simulink model "Model_Simulation"  (R2016a)
settings: Solver=FixedStepAuto  StartTime=0.0  StopTime=5  FixedStep=2e-6  RelTol=1e-3
values from neighbouring files (symbols this model uses):
  C = 3060e-6    (= 0.00306)    [Controle_Inversor_UR_D.m]
  Ki_i_disc = wc*Rf    (= 44.2477838534)    [Controle_Inversor_UR_D.m]
  Ki_i_disc_b = wc_b*Rb/Vdc    (= 0.0983284085631)    [Controle_Inversor_UR_D.m]
  Ki_q_disc = wq/H    [Controle_Inversor_UR_D.m]
  Ki_v_disc_b = wc_bv/Req    (= 14.5799013102)    [Controle_Inversor_UR_D.m]
  Ki_vdc_disc = ((wvdc)^2*C)/Gt    [Controle_Inversor_UR_D.m]
  Kp_i_disc = wc*Lf    (= 2.19688771906)    [Controle_Inversor_UR_D.m]
  Kp_i_disc_b = wc_b*Lb/Vdc    (= 0.00545604673435)    [Controle_Inversor_UR_D.m]
  Kp_q_disc = Ki_q_disc*(Lf/Kp_i_disc)    [Controle_Inversor_UR_D.m]
  Kp_v_disc_b = wc_bv*Cin    (= 0.0356301510224)    [Controle_Inversor_UR_D.m]
  Kp_vdc_disc = (2*ksi_vdc*wvdc*C)/Gt    [Controle_Inversor_UR_D.m]
  Lf = (0.0012+2.8949e-04)    (= 0.00148949)    [Controle_Inversor_UR_D.m]
  Tsw = 1/fsw    (= 0.0002)    [Controle_Inversor_UR_D.m]
  w = 2*pi*60    (= 376.991118431)    [Controle_Inversor_UR_D.m]
undefined symbols (not defined in the file or in its folder): D1, dEgdT, Delta, EgRef, gcbh, k1, Rsh_array5pc, sigbuilder_block, sps_rtmsupport, Tref_K, VT_ref
libraries: powerlib x179, simulink x14, powerlib_meascontrol x13, spsPVarrayModel x12
(part 20 of 20)

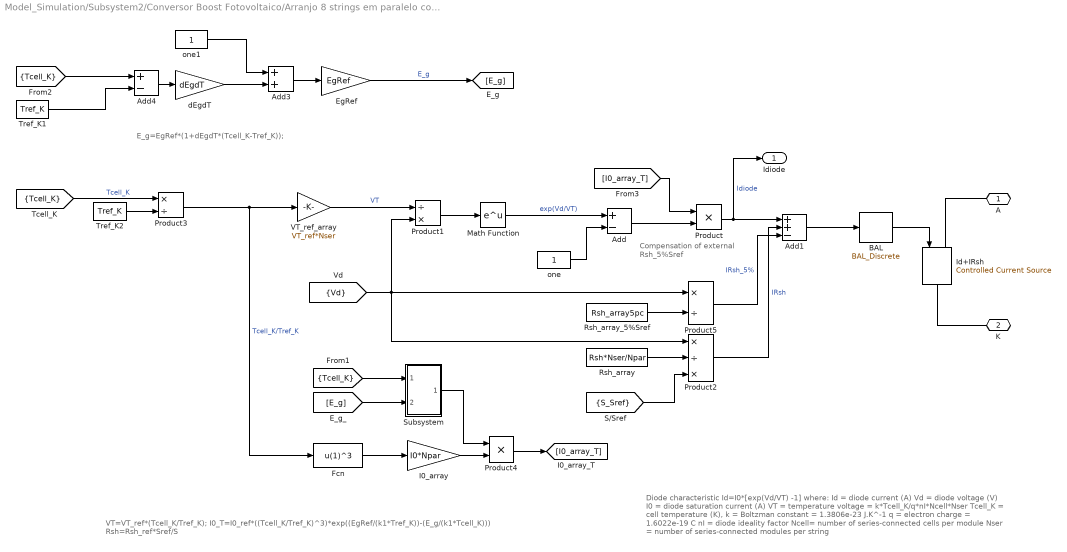
== system Model_Simulation/Subsystem2/Conversor Boost Fotovoltaico/Arranjo 8 strings em paralelo com 43 módulos em série Vmp = 43 x 30,6 = 1315,8 V Imp = 8,32 x 7 = 58,24 A 76.632,192 W/Diode Rsh ==
  note: E_g=EgRef*(1+dEgdT*(Tcell_K-Tref_K));
  note: VT=VT_ref*(Tcell_K/Tref_K);
      | I0_T=I0_ref*((Tcell_K/Tref_K)^3)*exp((EgRef/(k1*Tref_K))-(E_g/(k1*Tcell_K)))
      | Rsh=Rsh_ref*Sref/S
  note: Diode characteristic
      |    Id=I0*[exp(Vd/VT) -1]
      |
      | where:
      |      Id = diode current (A)
      |      Vd = diode voltage (V)
      |      I0 = diode saturation current (A)
      |      VT = temperature voltage = k*Tcell_K/q*nI*Ncell*Nser
      | Tcell_K = cell temperature (K),
      |       k = Boltzman constant = 1.3806e-23 J.K^-1
      |       q = electron charge = 1.6022e-19 C
      |      nI = diode ideality factor
      |    Ncell= number of series-connected cells per module
      |    Nser = number of series-connected modules per string
  note: Compensation of
      | external Rsh_5%Sref
  Add : Sum  Inputs=+-
  Add1 : Sum  Inputs=++-
  Add3 : Sum
  Add4 : Sum  Inputs=+-
  BAL : spsPVarrayModel/BAL_Discrete  VariantControl=NoBAL
  EgRef : Gain  Gain=EgRef
  Fcn : Fcn  Expr=u(1)^3
  I0_array : Gain  Gain=I0*Npar
  Id+IRsh : powerlib/Electrical Sources/Controlled Current Source  Initialize=on  Source_Type=AC  Amplitude=0  Phase=0  Frequency=0  Measurements=None
  Math Function : Math  SaturateOnIntegerOverflow=on
  Product : Product  RndMeth=Zero
  Product1 : Product  Inputs=/*  RndMeth=Zero
  Product2 : Product  Inputs=*/*  RndMeth=Zero
  Product3 : Product  Inputs=*/  RndMeth=Zero
  Product4 : Product  Inputs=**  RndMeth=Zero
  Product5 : Product  Inputs=*/  RndMeth=Zero
  Rsh_array : Constant  Value=Rsh*Nser/Npar
  Rsh_array_5%Sref : Constant  Value=Rsh_array5pc
  Subsystem : Subsystem
  Tref_K1 : Constant  Value=Tref_K
  Tref_K2 : Constant  Value=Tref_K
  VT_ref_array : Gain  Gain=VT_ref*Nser
  dEgdT : Gain  Gain=dEgdT
  one : Constant
  one1 : Constant
  A : PMIOPort  Port=1  Side=Left
  K : PMIOPort  Port=2  Side=Right
  Idiode : Outport
  wires:
  [Vd] -> Product1/2, Product2/1, Product5/1
  [S_Sref] -> Product2/3
  [I0_array_T] -> Product/1
  VT_ref_array/1 -> Product1/1  "VT"
  Add/1 -> Product/2
  Product4/1 -> [I0_array_T]
  Tref_K2/1 -> Product3/2
  [E_g] -> Subsystem/2(E_g)
  [Tcell_K] -> Subsystem/1(Tcell_K)
  Subsystem/1(exp) -> Product4/1
  Tref_K1/1 -> Add4/2
  [Tcell_K] -> Add4/1
  Fcn/1 -> I0_array/1
  I0_array/1 -> Product4/2
  EgRef/1 -> [E_g]  "E_g"
  Add3/1 -> EgRef/1
  dEgdT/1 -> Add3/2
  Add4/1 -> dEgdT/1
  one1/1 -> Add3/1
  Product3/1 -> Fcn/1, VT_ref_array/1  "Tcell_K/Tref_K"
  [Tcell_K] -> Product3/1  "Tcell_K"
  Rsh_array/1 -> Product2/2
  one/1 -> Add/2
  Product1/1 -> Math Function/1
  Product/1 -> Idiode/1, Add1/1  "Idiode"
  Product2/1 -> Add1/2  "IRsh"
  Math Function/1 -> Add/1  "exp(Vd/VT)"
  Rsh_array_5%Sref/1 -> Product5/2
  Product5/1 -> Add1/3  "IRsh_5%"
  Add1/1 -> BAL/1
  BAL/1 -> Id+IRsh/1
  connections:
  A/RConn1 -- Id+IRsh/LConn1
  Id+IRsh/RConn1 -- K/RConn1

== system Model_Simulation/Subsystem2/Conversor Boost Fotovoltaico/Arranjo 8 strings em paralelo com 43 módulos em série Vmp = 43 x 30,6 = 1315,8 V Imp = 8,32 x 7 = 58,24 A 76.632,192 W/IL ctrl ==
  note: IL=S/Sref*(IL_ref+alpha_isc*(Tcell_K-Tref_K));
  Temperature : Inport
  Irradiance : Inport  Port=2
  0_K : Constant  Value=273.15
  1/Sref : Gain  Gain=1e-3
  Add : Sum
  Add2 : Sum
  Add3 : Sum  Inputs=+-
  IL_module : Constant  Value=IL
  Npar : Gain  Gain=Npar
  Product1 : Product  Inputs=**  RndMeth=Zero
  Tref_K : Constant  Value=Tref_K
  alpha_Isc : Gain  Gain=alpha_Isc
  IL : Outport
  tag scope: S_Sref=scoped, Tcell_K=scoped
  wires:
  1/Sref/1 -> [S_Sref], Product1/2  "S/Sref"
  Npar/1 -> Product1/1
  Add2/1 -> [Tcell_K], Add3/1  "Tcell_K"
  Add/1 -> Npar/1
  0_K/1 -> Add2/2
  IL_module/1 -> Add/2
  Product1/1 -> IL/1  "IL"
  Tref_K/1 -> Add3/2
  Add3/1 -> alpha_Isc/1
  alpha_Isc/1 -> Add/1
  Irradiance/1 -> 1/Sref/1
  Temperature/1 -> Add2/1

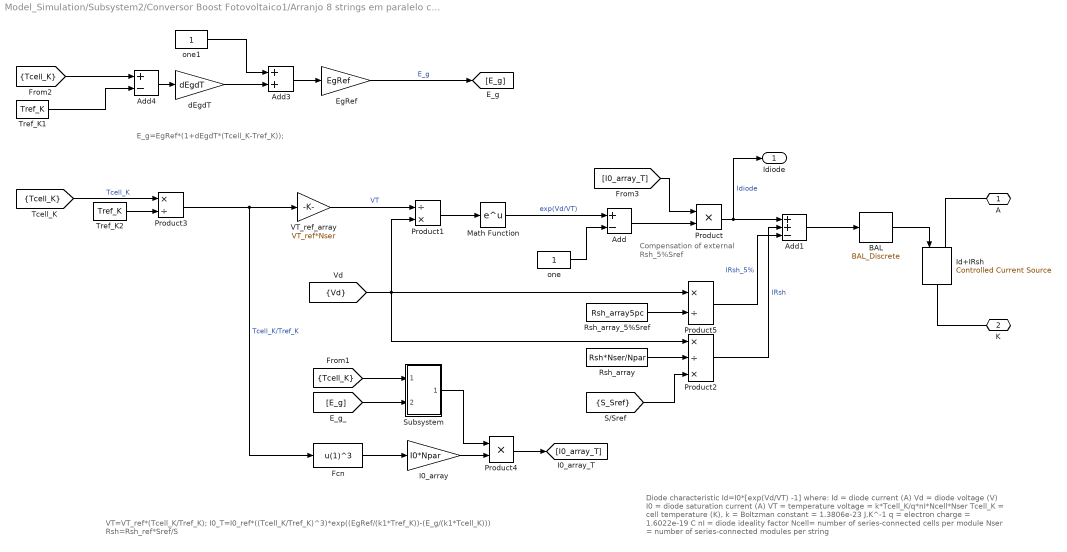
== system Model_Simulation/Subsystem2/Conversor Boost Fotovoltaico1/Arranjo 8 strings em paralelo com 43 módulos em série Vmp = 43 x 30,6 = 1315,8 V Imp = 8,32 x 7 = 58,24 A 76.632,192 W/Diode Rsh ==
  note: Compensation of
      | external Rsh_5%Sref
  note: Diode characteristic
      |    Id=I0*[exp(Vd/VT) -1]
      |
      | where:
      |      Id = diode current (A)
      |      Vd = diode voltage (V)
      |      I0 = diode saturation current (A)
      |      VT = temperature voltage = k*Tcell_K/q*nI*Ncell*Nser
      | Tcell_K = cell temperature (K),
      |       k = Boltzman constant = 1.3806e-23 J.K^-1
      |       q = electron charge = 1.6022e-19 C
      |      nI = diode ideality factor
      |    Ncell= number of series-connected cells per module
      |    Nser = number of series-connected modules per string
  note: VT=VT_ref*(Tcell_K/Tref_K);
      | I0_T=I0_ref*((Tcell_K/Tref_K)^3)*exp((EgRef/(k1*Tref_K))-(E_g/(k1*Tcell_K)))
      | Rsh=Rsh_ref*Sref/S
  note: E_g=EgRef*(1+dEgdT*(Tcell_K-Tref_K));
  Add : Sum  Inputs=+-
  Add1 : Sum  Inputs=++-
  Add3 : Sum
  Add4 : Sum  Inputs=+-
  BAL : spsPVarrayModel/BAL_Discrete  VariantControl=NoBAL
  EgRef : Gain  Gain=EgRef
  Fcn : Fcn  Expr=u(1)^3
  I0_array : Gain  Gain=I0*Npar
  Id+IRsh : powerlib/Electrical Sources/Controlled Current Source  Initialize=on  Source_Type=AC  Amplitude=0  Phase=0  Frequency=0  Measurements=None
  Math Function : Math  SaturateOnIntegerOverflow=on
  Product : Product  RndMeth=Zero
  Product1 : Product  Inputs=/*  RndMeth=Zero
  Product2 : Product  Inputs=*/*  RndMeth=Zero
  Product3 : Product  Inputs=*/  RndMeth=Zero
  Product4 : Product  Inputs=**  RndMeth=Zero
  Product5 : Product  Inputs=*/  RndMeth=Zero
  Rsh_array : Constant  Value=Rsh*Nser/Npar
  Rsh_array_5%Sref : Constant  Value=Rsh_array5pc
  Subsystem : Subsystem
  Tref_K1 : Constant  Value=Tref_K
  Tref_K2 : Constant  Value=Tref_K
  VT_ref_array : Gain  Gain=VT_ref*Nser
  dEgdT : Gain  Gain=dEgdT
  one : Constant
  one1 : Constant
  A : PMIOPort  Port=1  Side=Left
  K : PMIOPort  Port=2  Side=Right
  Idiode : Outport
  wires:
  BAL/1 -> Id+IRsh/1
  Add1/1 -> BAL/1
  Product5/1 -> Add1/3  "IRsh_5%"
  Rsh_array_5%Sref/1 -> Product5/2
  Math Function/1 -> Add/1  "exp(Vd/VT)"
  Product2/1 -> Add1/2  "IRsh"
  Product/1 -> Add1/1, Idiode/1  "Idiode"
  Product1/1 -> Math Function/1
  one/1 -> Add/2
  Rsh_array/1 -> Product2/2
  [Tcell_K] -> Product3/1  "Tcell_K"
  Product3/1 -> VT_ref_array/1, Fcn/1  "Tcell_K/Tref_K"
  one1/1 -> Add3/1
  Add4/1 -> dEgdT/1
  dEgdT/1 -> Add3/2
  Add3/1 -> EgRef/1
  EgRef/1 -> [E_g]  "E_g"
  I0_array/1 -> Product4/2
  Fcn/1 -> I0_array/1
  [Tcell_K] -> Add4/1
  Tref_K1/1 -> Add4/2
  Subsystem/1(exp) -> Product4/1
  [Tcell_K] -> Subsystem/1(Tcell_K)
  [E_g] -> Subsystem/2(E_g)
  Tref_K2/1 -> Product3/2
  Product4/1 -> [I0_array_T]
  Add/1 -> Product/2
  VT_ref_array/1 -> Product1/1  "VT"
  [I0_array_T] -> Product/1
  [S_Sref] -> Product2/3
  [Vd] -> Product5/1, Product2/1, Product1/2
  connections:
  Id+IRsh/RConn1 -- K/RConn1
  A/RConn1 -- Id+IRsh/LConn1

== system Model_Simulation/Subsystem2/Conversor Boost Fotovoltaico1/Arranjo 8 strings em paralelo com 43 módulos em série Vmp = 43 x 30,6 = 1315,8 V Imp = 8,32 x 7 = 58,24 A 76.632,192 W/IL ctrl ==
  note: IL=S/Sref*(IL_ref+alpha_isc*(Tcell_K-Tref_K));
  Temperature : Inport
  Irradiance : Inport  Port=2
  0_K : Constant  Value=273.15
  1/Sref : Gain  Gain=1e-3
  Add : Sum
  Add2 : Sum
  Add3 : Sum  Inputs=+-
  IL_module : Constant  Value=IL
  Npar : Gain  Gain=Npar
  Product1 : Product  Inputs=**  RndMeth=Zero
  Tref_K : Constant  Value=Tref_K
  alpha_Isc : Gain  Gain=alpha_Isc
  IL : Outport
  tag scope: S_Sref=scoped, Tcell_K=scoped
  wires:
  Temperature/1 -> Add2/1
  Irradiance/1 -> 1/Sref/1
  alpha_Isc/1 -> Add/1
  Add3/1 -> alpha_Isc/1
  Tref_K/1 -> Add3/2
  Product1/1 -> IL/1  "IL"
  IL_module/1 -> Add/2
  0_K/1 -> Add2/2
  Add/1 -> Npar/1
  Add2/1 -> Add3/1, [Tcell_K]  "Tcell_K"
  Npar/1 -> Product1/1
  1/Sref/1 -> Product1/2, [S_Sref]  "S/Sref"

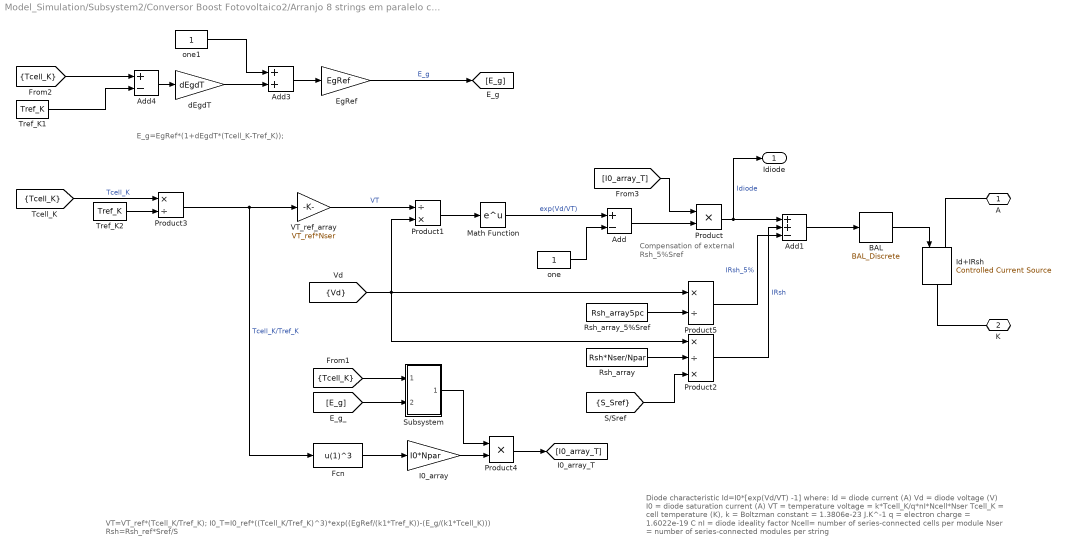
== system Model_Simulation/Subsystem2/Conversor Boost Fotovoltaico2/Arranjo 8 strings em paralelo com 43 módulos em série Vmp = 43 x 30,6 = 1315,8 V Imp = 8,32 x 7 = 58,24 A 76.632,192 W/Diode Rsh ==
  note: E_g=EgRef*(1+dEgdT*(Tcell_K-Tref_K));
  note: VT=VT_ref*(Tcell_K/Tref_K);
      | I0_T=I0_ref*((Tcell_K/Tref_K)^3)*exp((EgRef/(k1*Tref_K))-(E_g/(k1*Tcell_K)))
      | Rsh=Rsh_ref*Sref/S
  note: Diode characteristic
      |    Id=I0*[exp(Vd/VT) -1]
      |
      | where:
      |      Id = diode current (A)
      |      Vd = diode voltage (V)
      |      I0 = diode saturation current (A)
      |      VT = temperature voltage = k*Tcell_K/q*nI*Ncell*Nser
      | Tcell_K = cell temperature (K),
      |       k = Boltzman constant = 1.3806e-23 J.K^-1
      |       q = electron charge = 1.6022e-19 C
      |      nI = diode ideality factor
      |    Ncell= number of series-connected cells per module
      |    Nser = number of series-connected modules per string
  note: Compensation of
      | external Rsh_5%Sref
  Add : Sum  Inputs=+-
  Add1 : Sum  Inputs=++-
  Add3 : Sum
  Add4 : Sum  Inputs=+-
  BAL : spsPVarrayModel/BAL_Discrete  VariantControl=NoBAL
  EgRef : Gain  Gain=EgRef
  Fcn : Fcn  Expr=u(1)^3
  I0_array : Gain  Gain=I0*Npar
  Id+IRsh : powerlib/Electrical Sources/Controlled Current Source  Initialize=on  Source_Type=AC  Amplitude=0  Phase=0  Frequency=0  Measurements=None
  Math Function : Math  SaturateOnIntegerOverflow=on
  Product : Product  RndMeth=Zero
  Product1 : Product  Inputs=/*  RndMeth=Zero
  Product2 : Product  Inputs=*/*  RndMeth=Zero
  Product3 : Product  Inputs=*/  RndMeth=Zero
  Product4 : Product  Inputs=**  RndMeth=Zero
  Product5 : Product  Inputs=*/  RndMeth=Zero
  Rsh_array : Constant  Value=Rsh*Nser/Npar
  Rsh_array_5%Sref : Constant  Value=Rsh_array5pc
  Subsystem : Subsystem
  Tref_K1 : Constant  Value=Tref_K
  Tref_K2 : Constant  Value=Tref_K
  VT_ref_array : Gain  Gain=VT_ref*Nser
  dEgdT : Gain  Gain=dEgdT
  one : Constant
  one1 : Constant
  A : PMIOPort  Port=1  Side=Left
  K : PMIOPort  Port=2  Side=Right
  Idiode : Outport
  wires:
  [Vd] -> Product1/2, Product2/1, Product5/1
  [S_Sref] -> Product2/3
  [I0_array_T] -> Product/1
  VT_ref_array/1 -> Product1/1  "VT"
  Add/1 -> Product/2
  Product4/1 -> [I0_array_T]
  Tref_K2/1 -> Product3/2
  [E_g] -> Subsystem/2(E_g)
  [Tcell_K] -> Subsystem/1(Tcell_K)
  Subsystem/1(exp) -> Product4/1
  Tref_K1/1 -> Add4/2
  [Tcell_K] -> Add4/1
  Fcn/1 -> I0_array/1
  I0_array/1 -> Product4/2
  EgRef/1 -> [E_g]  "E_g"
  Add3/1 -> EgRef/1
  dEgdT/1 -> Add3/2
  Add4/1 -> dEgdT/1
  one1/1 -> Add3/1
  Product3/1 -> Fcn/1, VT_ref_array/1  "Tcell_K/Tref_K"
  [Tcell_K] -> Product3/1  "Tcell_K"
  Rsh_array/1 -> Product2/2
  one/1 -> Add/2
  Product1/1 -> Math Function/1
  Product/1 -> Idiode/1, Add1/1  "Idiode"
  Product2/1 -> Add1/2  "IRsh"
  Math Function/1 -> Add/1  "exp(Vd/VT)"
  Rsh_array_5%Sref/1 -> Product5/2
  Product5/1 -> Add1/3  "IRsh_5%"
  Add1/1 -> BAL/1
  BAL/1 -> Id+IRsh/1
  connections:
  A/RConn1 -- Id+IRsh/LConn1
  Id+IRsh/RConn1 -- K/RConn1

== system Model_Simulation/Subsystem2/Conversor Boost Fotovoltaico2/Arranjo 8 strings em paralelo com 43 módulos em série Vmp = 43 x 30,6 = 1315,8 V Imp = 8,32 x 7 = 58,24 A 76.632,192 W/IL ctrl ==
  note: IL=S/Sref*(IL_ref+alpha_isc*(Tcell_K-Tref_K));
  Temperature : Inport
  Irradiance : Inport  Port=2
  0_K : Constant  Value=273.15
  1/Sref : Gain  Gain=1e-3
  Add : Sum
  Add2 : Sum
  Add3 : Sum  Inputs=+-
  IL_module : Constant  Value=IL
  Npar : Gain  Gain=Npar
  Product1 : Product  Inputs=**  RndMeth=Zero
  Tref_K : Constant  Value=Tref_K
  alpha_Isc : Gain  Gain=alpha_Isc
  IL : Outport
  tag scope: S_Sref=scoped, Tcell_K=scoped
  wires:
  1/Sref/1 -> [S_Sref], Product1/2  "S/Sref"
  Npar/1 -> Product1/1
  Add2/1 -> [Tcell_K], Add3/1  "Tcell_K"
  Add/1 -> Npar/1
  0_K/1 -> Add2/2
  IL_module/1 -> Add/2
  Product1/1 -> IL/1  "IL"
  Tref_K/1 -> Add3/2
  Add3/1 -> alpha_Isc/1
  alpha_Isc/1 -> Add/1
  Irradiance/1 -> 1/Sref/1
  Temperature/1 -> Add2/1

== system Model_Simulation/Subsystem2/Conversor Boost Fotovoltaico/Arranjo 8 strings em paralelo com 43 módulos em série Vmp = 43 x 30,6 = 1315,8 V Imp = 8,32 x 7 = 58,24 A 76.632,192 W/Diode Rsh/Subsystem ==
  note: exp((EgRef/(k1*Tref_K))-(E_g/(k1*Tcell_K)))
  Tcell_K : Inport
  E_g : Inport  Port=2
  Add : Sum  Inputs=+-
  EgRef : Constant  Value=EgRef/(k1*Tref_K)
  Math Function : Math  SaturateOnIntegerOverflow=on
  Product : Product  Inputs=*/
  k1 : Gain  Gain=k1
  exp : Outport
  wires:
  Math Function/1 -> exp/1
  Add/1 -> Math Function/1
  Product/1 -> Add/2
  k1/1 -> Product/2
  Tcell_K/1 -> k1/1
  E_g/1 -> Product/1
  EgRef/1 -> Add/1

== system Model_Simulation/Subsystem2/Conversor Boost Fotovoltaico1/Arranjo 8 strings em paralelo com 43 módulos em série Vmp = 43 x 30,6 = 1315,8 V Imp = 8,32 x 7 = 58,24 A 76.632,192 W/Diode Rsh/Subsystem ==
  note: exp((EgRef/(k1*Tref_K))-(E_g/(k1*Tcell_K)))
  Tcell_K : Inport
  E_g : Inport  Port=2
  Add : Sum  Inputs=+-
  EgRef : Constant  Value=EgRef/(k1*Tref_K)
  Math Function : Math  SaturateOnIntegerOverflow=on
  Product : Product  Inputs=*/
  k1 : Gain  Gain=k1
  exp : Outport
  wires:
  EgRef/1 -> Add/1
  E_g/1 -> Product/1
  Tcell_K/1 -> k1/1
  k1/1 -> Product/2
  Product/1 -> Add/2
  Add/1 -> Math Function/1
  Math Function/1 -> exp/1

== system Model_Simulation/Subsystem2/Conversor Boost Fotovoltaico2/Arranjo 8 strings em paralelo com 43 módulos em série Vmp = 43 x 30,6 = 1315,8 V Imp = 8,32 x 7 = 58,24 A 76.632,192 W/Diode Rsh/Subsystem ==
  note: exp((EgRef/(k1*Tref_K))-(E_g/(k1*Tcell_K)))
  Tcell_K : Inport
  E_g : Inport  Port=2
  Add : Sum  Inputs=+-
  EgRef : Constant  Value=EgRef/(k1*Tref_K)
  Math Function : Math  SaturateOnIntegerOverflow=on
  Product : Product  Inputs=*/
  k1 : Gain  Gain=k1
  exp : Outport
  wires:
  Math Function/1 -> exp/1
  Add/1 -> Math Function/1
  Product/1 -> Add/2
  k1/1 -> Product/2
  Tcell_K/1 -> k1/1
  E_g/1 -> Product/1
  EgRef/1 -> Add/1

== matlab function Model_Simulation/Subsystem2/ABC2DQ3/Transformada de Clarke abc para alfa_beta_zero ==
  data: fa input; falfa output; fb input; fc input; fbeta output; fzero output
function [falfa,fbeta,fzero] = fcn(fa, fb, fc)
%#codegen
k = 2/3;

falfa = k*(  1*fa -         0.5*fb -         0.5*fc);
fbeta = k*(  0*fa + (sqrt(3)/2)*fb - (sqrt(3)/2)*fc);
fzero = k*(0.5*fa +         0.5*fb +         0.5*fc);

== matlab function Model_Simulation/Subsystem2/ABC2DQ3/Transformada de Park alfa_beta_zero para dq0 ==
  data: falfa input; fbeta input; fzero input; fd output; fq output; f0 output; theta input
function [fd,fq,f0] = fcn(falfa, fbeta, fzero, theta)
%#codegen
fd = ( cos(theta)*falfa + sin(theta)*fbeta + 0*fzero);
fq = (-sin(theta)*falfa + cos(theta)*fbeta + 0*fzero);
f0 = fzero;

== matlab function Model_Simulation/Subsystem2/MPPT e controle Boost1/AVR antigo/MATLAB Function ==
  data: u input; y output
function y = fcn(u)

if u>=3.1
    y = 0.33
elseif u<=2.3
    y = 0.1
else
    y = u
end

== matlab function Model_Simulation/Subsystem2/MPPT e controle Boost1/MATLAB Function ==
  data: Vpv input; Ipv input; Vref output; MO input; S input
function Vref  = PeO(Vpv,Ipv,MO,S)
persistent Vpv_old
persistent Ppv_old
persistent Vpv_ref
persistent sinal
persistent Vinc
persistent Ppv_trav

if isempty(Vpv_old)
    Vpv_old = 0;
end
if isempty(Ppv_old)
    Ppv_old = 0;
end
if isempty(Vpv_ref)
    Vpv_ref = 1316;
end
if isempty(sinal)
    sinal = 0;
end
if isempty(Vinc)
    Vinc = 1;
end
if isempty(Ppv_trav)
    Ppv_trav = 0;
end

if MO <1
    Vref = Vpv_ref;
    if sinal == 1
        Vinc = 20;
        if Vref > 1300
            sinal = 0;
            Vinc = 1;
        else
            Vref = Vref + Vinc;
        end
    end
Ppv = Vpv*Ipv;
del_Ppv = Ppv - Ppv_old;
del_Vpv = Vpv - Vpv_old;

if(del_Ppv > 0 && sinal == 0)
    if(del_Vpv > 0)
        Vref = Vref + Vinc;
    else
        Vref = Vref - Vinc;
    end
end

if(del_Ppv < 0 && sinal == 0)
    if(del_Vpv > 0)
        Vref = Vref - Vinc;
    else
        Vref = Vref + Vinc;
    end
end

Ppv_old = Ppv;
Vpv_old = Vpv;
Vpv_ref = Vref;
end

if MO >= 1
Ppv = Vpv*Ipv;
    if sinal <= 0
        Ppv_trav = Ppv;
        sinal = 1;
        Vinc = 20;
    end
    Vref = Vpv_ref;
    Ppv_set = Ppv_trav*S;
if (Ppv > Ppv_set)
    if(Ppv > 20000)
        Vref = Vpv_ref - Vinc;
    else
        Vref = Vpv_ref;
    end
end
Ppv_old = Ppv;
Vpv_old = Vpv;
Vpv_ref = Vref;
else
    Vref = Vpv_ref;
end
end

== matlab function Model_Simulation/Subsystem2/Controle do inversor/DQ0toABC/Transformada de Clarke alfa_beta_zero para abc ==
  data: fa output; falfa input; fb output; fc output; fbeta input; fzero input
function [fa,fb,fc] = fcn(falfa, fbeta, fzero)
%#codegen
fa = (   1*falfa +           0*fbeta + 1*fzero);
fb = (-0.5*falfa + (sqrt(3)/2)*fbeta + 1*fzero);
fc = (-0.5*falfa - (sqrt(3)/2)*fbeta + 1*fzero);

== matlab function Model_Simulation/Subsystem2/Controle do inversor/DQ0toABC/Transformada de Park dq0 para alfa_beta_zero ==
  data: falfa output; fbeta output; fzero output; fd input; fq input; f0 input; theta input
function [falfa,fbeta,fzero] = fcn(fd, fq, f0, theta)
%#codegen
falfa = (cos(theta)*fd - sin(theta)*fq + 0*f0);
fbeta = (sin(theta)*fd + cos(theta)*fq + 0*f0);
fzero = f0;

== matlab function Model_Simulation/Subsystem2/ABC2DQ/Transformada de Clarke abc para alfa_beta_zero ==
  data: fa input; falfa output; fb input; fc input; fbeta output; fzero output
function [falfa,fbeta,fzero] = fcn(fa, fb, fc)
%#codegen
k = 2/3;

falfa = k*(  1*fa -         0.5*fb -         0.5*fc);
fbeta = k*(  0*fa + (sqrt(3)/2)*fb - (sqrt(3)/2)*fc);
fzero = k*(0.5*fa +         0.5*fb +         0.5*fc);

== matlab function Model_Simulation/Subsystem2/ABC2DQ/Transformada de Park alfa_beta_zero para dq0 ==
  data: falfa input; fbeta input; fzero input; fd output; fq output; f0 output; theta input
function [fd,fq,f0] = fcn(falfa, fbeta, fzero, theta)
%#codegen
fd = ( cos(theta)*falfa + sin(theta)*fbeta + 0*fzero);
fq = (-sin(theta)*falfa + cos(theta)*fbeta + 0*fzero);
f0 = fzero;

== matlab function Model_Simulation/Subsystem2/MPPT e controle Boost1/MATLAB Function1 ==
  data: Vpv input; Ipv input; Vref output
function Vref = PeO(Vpv,Ipv)
persistent Vpv_old
persistent Ppv_old
persistent Vpv_ref
Vinc = 0.1;

if isempty(Vpv_old)
    Vpv_old = 0;
end
if isempty(Ppv_old)
    Ppv_old = 0;
end
if isempty(Vpv_ref)
    Vpv_ref = 1102;
end

Vref = Vpv_ref;
Ppv = Vpv*Ipv;
del_Ppv = Ppv - Ppv_old;
del_Vpv = Vpv - Vpv_old;

if(del_Ppv > 0)
    if(del_Vpv > 0)
        Vref = Vref + Vinc;
    else
        Vref = Vref - Vinc;
    end
end

if(del_Ppv < 0)
    if(del_Vpv > 0)
        Vref = Vref - Vinc;
    else
        Vref = Vref + Vinc;
    end
end

Ppv_old = Ppv;
Vpv_old = Vpv;
Vpv_ref = Vref;
end

== matlab function Model_Simulation/Subsystem2/MPPT e controle Boost2/MATLAB Function ==
  data: Vpv input; Ipv input; Vref output; MO input; S input
function Vref  = PeO(Vpv,Ipv,MO,S)
persistent Vpv_old
persistent Ppv_old
persistent Vpv_ref
persistent sinal
persistent Vinc
persistent Ppv_trav

if isempty(Vpv_old)
    Vpv_old = 0;
end
if isempty(Ppv_old)
    Ppv_old = 0;
end
if isempty(Vpv_ref)
    Vpv_ref = 1316;
end
if isempty(sinal)
    sinal = 0;
end
if isempty(Vinc)
    Vinc = 1;
end
if isempty(Ppv_trav)
    Ppv_trav = 0;
end

if MO <1
    Vref = Vpv_ref;
    if sinal == 1
        Vinc = 20;
        if Vref > 1300
            sinal = 0;
            Vinc = 1;
        else
            Vref = Vref + Vinc;
        end
    end
Ppv = Vpv*Ipv;
del_Ppv = Ppv - Ppv_old;
del_Vpv = Vpv - Vpv_old;

if(del_Ppv > 0 && sinal == 0)
    if(del_Vpv > 0)
        Vref = Vref + Vinc;
    else
        Vref = Vref - Vinc;
    end
end

if(del_Ppv < 0 && sinal == 0)
    if(del_Vpv > 0)
        Vref = Vref - Vinc;
    else
        Vref = Vref + Vinc;
    end
end

Ppv_old = Ppv;
Vpv_old = Vpv;
Vpv_ref = Vref;
end

if MO >= 1
Ppv = Vpv*Ipv;
    if sinal <= 0
        Ppv_trav = Ppv;
        sinal = 1;
        Vinc = 20;
    end
    Vref = Vpv_ref;
    Ppv_set = Ppv_trav*S;
if (Ppv > Ppv_set)
    if(Ppv > 20000)
        Vref = Vpv_ref - Vinc;
    else
        Vref = Vpv_ref;
    end
end
Ppv_old = Ppv;
Vpv_old = Vpv;
Vpv_ref = Vref;
else
    Vref = Vpv_ref;
end
end

== matlab function Model_Simulation/Subsystem2/MPPT e controle Boost2/MATLAB Function1 ==
  data: Vpv input; Ipv input; Vref output
function Vref = PeO(Vpv,Ipv)
persistent Vpv_old
persistent Ppv_old
persistent Vpv_ref
Vinc = 0.1;

if isempty(Vpv_old)
    Vpv_old = 0;
end
if isempty(Ppv_old)
    Ppv_old = 0;
end
if isempty(Vpv_ref)
    Vpv_ref = 1102;
end

Vref = Vpv_ref;
Ppv = Vpv*Ipv;
del_Ppv = Ppv - Ppv_old;
del_Vpv = Vpv - Vpv_old;

if(del_Ppv > 0)
    if(del_Vpv > 0)
        Vref = Vref + Vinc;
    else
        Vref = Vref - Vinc;
    end
end

if(del_Ppv < 0)
    if(del_Vpv > 0)
        Vref = Vref - Vinc;
    else
        Vref = Vref + Vinc;
    end
end

Ppv_old = Ppv;
Vpv_old = Vpv;
Vpv_ref = Vref;
end

== matlab function Model_Simulation/Subsystem2/MPPT e controle Boost3/MATLAB Function ==
  data: Vpv input; Ipv input; Vref output; MO input; S input
function Vref  = PeO(Vpv,Ipv,MO,S)
persistent Vpv_old
persistent Ppv_old
persistent Vpv_ref
persistent sinal
persistent Vinc
persistent Ppv_trav

if isempty(Vpv_old)
    Vpv_old = 0;
end
if isempty(Ppv_old)
    Ppv_old = 0;
end
if isempty(Vpv_ref)
    Vpv_ref = 1316;
end
if isempty(sinal)
    sinal = 0;
end
if isempty(Vinc)
    Vinc = 1;
end
if isempty(Ppv_trav)
    Ppv_trav = 0;
end

if MO <1
    Vref = Vpv_ref;
    if sinal == 1
        Vinc = 20;
        if Vref > 1300
            sinal = 0;
            Vinc = 1;
        else
            Vref = Vref + Vinc;
        end
    end
Ppv = Vpv*Ipv;
del_Ppv = Ppv - Ppv_old;
del_Vpv = Vpv - Vpv_old;

if(del_Ppv > 0 && sinal == 0)
    if(del_Vpv > 0)
        Vref = Vref + Vinc;
    else
        Vref = Vref - Vinc;
    end
end

if(del_Ppv < 0 && sinal == 0)
    if(del_Vpv > 0)
        Vref = Vref - Vinc;
    else
        Vref = Vref + Vinc;
    end
end

Ppv_old = Ppv;
Vpv_old = Vpv;
Vpv_ref = Vref;
end

if MO >= 1
Ppv = Vpv*Ipv;
    if sinal <= 0
        Ppv_trav = Ppv;
        sinal = 1;
        Vinc = 20;
    end
    Vref = Vpv_ref;
    Ppv_set = Ppv_trav*S;
if (Ppv > Ppv_set)
    if(Ppv > 20000)
        Vref = Vpv_ref - Vinc;
    else
        Vref = Vpv_ref;
    end
end
Ppv_old = Ppv;
Vpv_old = Vpv;
Vpv_ref = Vref;
else
    Vref = Vpv_ref;
end
end
